simulink model "SecondSimulinkProblem"  (R2020b)
settings: Solver=VariableStepAuto  StartTime=0.0  StopTime=10.0  RelTol=1e-3
libraries: simulink x2
settings Model: Creator=parke  LastModifiedBy=parke

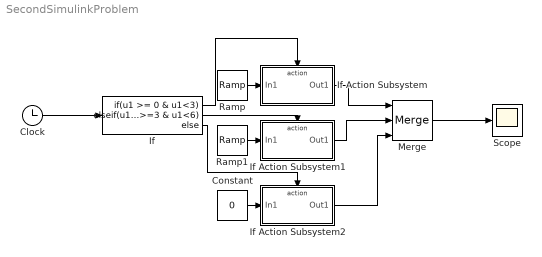
== system SecondSimulinkProblem ==
  Clock : Clock
  Constant : Constant  Value=0
  If : If  IfExpression=u1 >= 0 & u1<3  ElseIfExpressions=u1>=3 & u1<6
  If Action Subsystem : Subsystem  TreatAsAtomicUnit=on
  If Action Subsystem1 : Subsystem  TreatAsAtomicUnit=on
  If Action Subsystem2 : Subsystem  TreatAsAtomicUnit=on
  Merge : Merge  Inputs=3
  Ramp : simulink/Sources/Ramp  slope=1  start=0  InitialOutput=0
  Ramp1 : simulink/Sources/Ramp  slope=-1  start=0  InitialOutput=6
  Scope : Scope
  wires:
  Clock/1 -> If/1
  If/1 -> If Action Subsystem/Action
  If/2 -> If Action Subsystem1/Action
  If/3 -> If Action Subsystem2/Action
  Ramp/1 -> If Action Subsystem/1(In1)
  Ramp1/1 -> If Action Subsystem1/1(In1)
  Constant/1 -> If Action Subsystem2/1(In1)
  If Action Subsystem/1(Out1) -> Merge/1
  If Action Subsystem1/1(Out1) -> Merge/2
  If Action Subsystem2/1(Out1) -> Merge/3
  Merge/1 -> Scope/1

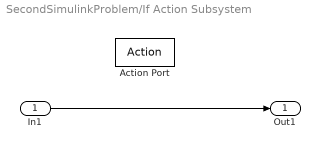
== system SecondSimulinkProblem/If Action Subsystem ==
  In1 : Inport
  Action Port : ActionPort  ActionPortLabel=if(u1 >= 0 & u1<3)
  Out1 : Outport
  wires:
  In1/1 -> Out1/1

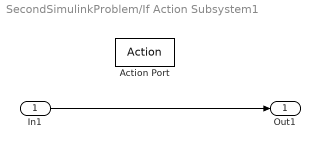
== system SecondSimulinkProblem/If Action Subsystem1 ==
  In1 : Inport
  Action Port : ActionPort  ActionPortLabel=elseif(u1>=3 & u1<6)
  Out1 : Outport
  wires:
  In1/1 -> Out1/1

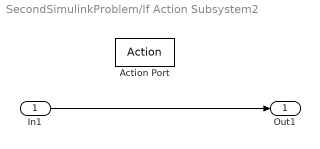
== system SecondSimulinkProblem/If Action Subsystem2 ==
  In1 : Inport
  Action Port : ActionPort  ActionPortLabel=else
  Out1 : Outport
  wires:
  In1/1 -> Out1/1
